simulink model "ModelTest"  (R2018b)
settings: Solver=ode1  StartTime=0.0  StopTime=50.0  FixedStep=0.001  RelTol=1e-3
undefined symbols (not defined in the file): env, sim, steer, vehicle
libraries: simulink x8, dspsrcs4 x1
settings Model: Creator=ogihara  LastModifiedBy=ogihara

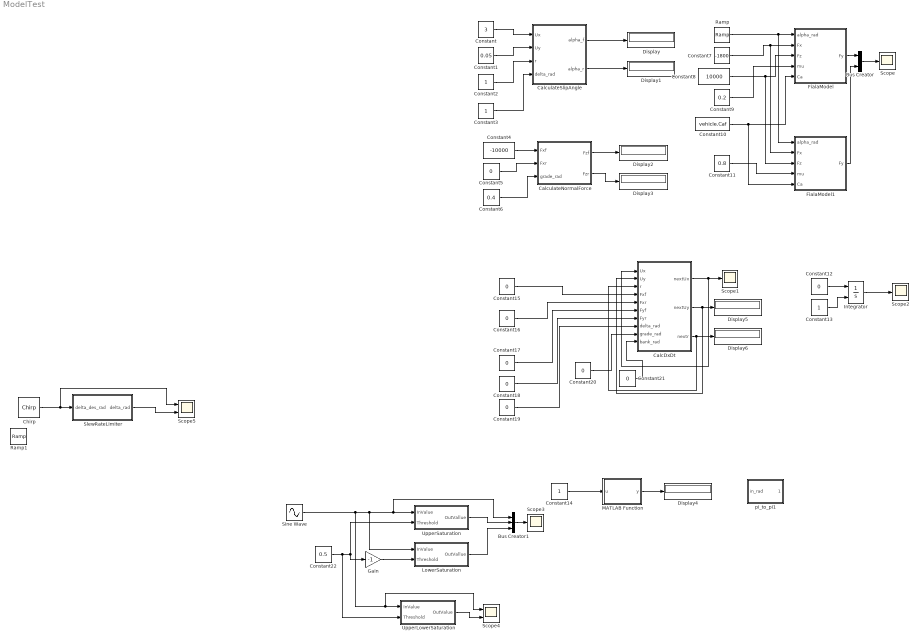
== system ModelTest ==
  Bus Creator : BusCreator  Inputs=2
  Bus Creator1 : BusCreator  Inputs=3
  CalcDxDt : Subsystem
  CalculateNormalForce : Subsystem
  CalculateSlipAngle : Subsystem
  Chirp : dspsrcs4/Chirp  sweep=Linear  mode=Unidirectional  f0=0.1  f1=1  t1=100  Tsweep=100  phase=0  Ts=1/1000  spf=1  datatype=Double  OutputFrames=off
      settings: SourceProductName=DSP System Toolbox
  Constant : Constant  Value=3
  Constant1 : Constant  Value=0.05
  Constant10 : Constant  Value=vehicle.Caf
  Constant11 : Constant  Value=0.8
  Constant{5,12,15..21} (9 alike) : Constant  Value=0
  Constant{2..3,13..14} (4 alike) : Constant
  Constant22 : Constant  Value=0.5
  Constant4 : Constant  Value=-10000
  Constant6 : Constant  Value=0.4
  Constant7 : Constant  Value=-1800
  Constant8 : Constant  Value=10000
  Constant9 : Constant  Value=0.2
  Display{,1..6} (7 alike) : Display
  FialaModel : Subsystem
  FialaModel1 : Subsystem
  Gain : Gain  Gain=-1
  Integrator : Integrator  InitialConditionSource=external
  LowerSaturation : Subsystem
  MATLAB Function : MATLAB Function  TreatAsAtomicUnit=on
  Ramp : simulink/Sources/Ramp  slope=0.1  start=0  InitialOutput=-0.5
  Ramp1 : simulink/Sources/Ramp  slope=1  start=0  InitialOutput=0
  Scope{,1..3} (4 alike) : Scope
  Scope4 : Scope  NumInputPorts=2
  Scope5 : Scope  NumInputPorts=2
  Sine Wave : Sin  SampleTime=0
  SlewRateLimiter : Subsystem
  UpperLowerSaturation : Subsystem
  UpperSaturation : Subsystem
  pi_to_pi1 : Subsystem
  wires:
  CalculateSlipAngle/2(alpha_r) -> Display1/1
  CalculateSlipAngle/1(alpha_f) -> Display/1
  Constant/1 -> CalculateSlipAngle/1(Ux)
  Constant1/1 -> CalculateSlipAngle/2(Uy)
  Constant2/1 -> CalculateSlipAngle/3(r)
  Constant3/1 -> CalculateSlipAngle/4(delta_rad)
  Constant4/1 -> CalculateNormalForce/1(Fxf)
  Constant5/1 -> CalculateNormalForce/2(Fxr)
  Constant6/1 -> CalculateNormalForce/3(grade_rad)
  CalculateNormalForce/1(Fzf) -> Display2/1
  CalculateNormalForce/2(Fzr) -> Display3/1
  Ramp/1 -> FialaModel1/1(alpha_rad), FialaModel/1(alpha_rad)
  Constant7/1 -> FialaModel1/2(Fx), FialaModel/2(Fx)
  Constant8/1 -> FialaModel1/3(Fz), FialaModel/3(Fz)
  Constant9/1 -> FialaModel/4(mu)
  Constant10/1 -> FialaModel1/5(Ca), FialaModel/5(Ca)
  Constant11/1 -> FialaModel1/4(mu)
  FialaModel/1(Fy) -> Bus Creator/1
  FialaModel1/1(Fy) -> Bus Creator/2
  Bus Creator/1 -> Scope/1
  Constant15/1 -> CalcDxDt/4(Fxf)
  Constant16/1 -> CalcDxDt/5(Fxr)
  Constant17/1 -> CalcDxDt/6(Fyf)
  Constant18/1 -> CalcDxDt/7(Fyr)
  Constant19/1 -> CalcDxDt/8(delta_rad)
  Constant21/1 -> CalcDxDt/10(bank_rad)
  Constant20/1 -> CalcDxDt/9(grade_rad)
  CalcDxDt/3(nextr) -> CalcDxDt/3(r), Display6/1
  CalcDxDt/2(nextUy) -> CalcDxDt/2(Uy), Display5/1
  CalcDxDt/1("nextUx ") -> CalcDxDt/1(Ux), Scope1/1
  Integrator/1 -> Scope2/1
  Constant13/1 -> Integrator/2
  Constant12/1 -> Integrator/1
  MATLAB Function/1(y) -> Display4/1
  Constant14/1 -> MATLAB Function/1(u)
  Sine Wave/1 -> Scope4/1, UpperLowerSaturation/1(InValue), LowerSaturation/1(InValue), Bus Creator1/1, UpperSaturation/1(InValue)
  Constant22/1 -> UpperLowerSaturation/2(Threshold), Gain/1, UpperSaturation/2(Threshold)
  Gain/1 -> LowerSaturation/2(Threshold)
  UpperSaturation/1(OutVallue) -> Bus Creator1/2
  LowerSaturation/1(OutVallue) -> Bus Creator1/3
  Bus Creator1/1 -> Scope3/1
  UpperLowerSaturation/1(OutValue) -> Scope4/2
  Chirp/1 -> Scope5/1, SlewRateLimiter/1(delta_des_rad)
  SlewRateLimiter/1(delta_rad) -> Scope5/2

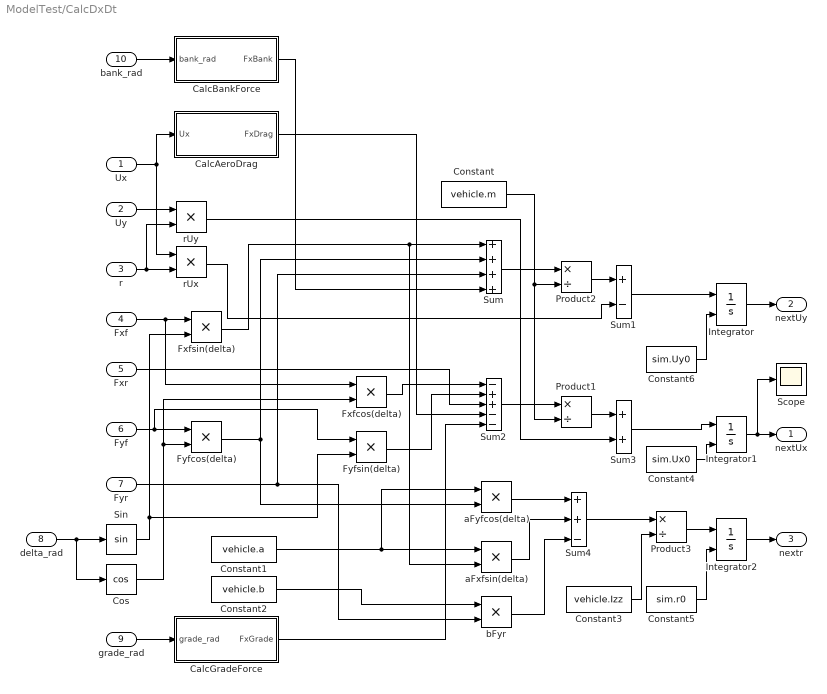
== system ModelTest/CalcDxDt ==
  Ux : Inport
  Uy : Inport  Port=2
  r : Inport  Port=3
  Fxf : Inport  Port=4
  Fxr : Inport  Port=5
  Fyf : Inport  Port=6
  Fyr : Inport  Port=7
  delta_rad : Inport  Port=8
  grade_rad : Inport  Port=9
  bank_rad : Inport  Port=10
  CalcAeroDrag : Subsystem
  CalcBankForce : Subsystem
  CalcGradeForce : Subsystem
  Constant : Constant  Value=vehicle.m
  Constant1 : Constant  Value=vehicle.a
  Constant2 : Constant  Value=vehicle.b
  Constant3 : Constant  Value=vehicle.Izz
  Constant4 : Constant  Value=sim.Ux0
  Constant5 : Constant  Value=sim.r0
  Constant6 : Constant  Value=sim.Uy0
  Cos : Trigonometry  Operator=cos
  Fxfcos(delta) : Product
  Fxfsin(delta) : Product
  Fyfcos(delta) : Product
  Fyfsin(delta) : Product
  Integrator : Integrator  InitialConditionSource=external
  Integrator1 : Integrator  InitialConditionSource=external
  Integrator2 : Integrator  InitialConditionSource=external  InitialCondition=sim.r0
  Product1 : Product  Inputs=*/
  Product2 : Product  Inputs=*/
  Product3 : Product  Inputs=*/
  Scope : Scope
  Sin : Trigonometry
  Sum : Sum  Inputs=++++
  Sum1 : Sum  Inputs=+-
  Sum2 : Sum  Inputs=-++--
  Sum3 : Sum
  Sum4 : Sum  Inputs=++-
  aFxfsin(delta) : Product
  aFyfcos(delta) : Product
  bFyr : Product
  rUx : Product
  rUy : Product
  "nextUx " : Outport
  nextUy : Outport  Port=2
  nextr : Outport  Port=3
  wires:
  delta_rad/1 -> Cos/1, Sin/1
  Fyf/1 -> Fyfsin(delta)/1, Fyfcos(delta)/1
  Cos/1 -> Fxfcos(delta)/2, Fyfcos(delta)/2
  Fxf/1 -> Fxfcos(delta)/1, Fxfsin(delta)/1
  Sin/1 -> Fyfsin(delta)/2, Fxfsin(delta)/2
  Fxfsin(delta)/1 -> Sum/1, aFxfsin(delta)/2
  Fyfcos(delta)/1 -> aFyfcos(delta)/2, Sum/2
  Fyr/1 -> bFyr/2, Sum/3
  grade_rad/1 -> CalcGradeForce/1(grade_rad)
  Constant/1 -> Product1/2, Product2/2
  Sum/1 -> Product2/1
  r/1 -> rUx/2, rUy/2
  Ux/1 -> CalcAeroDrag/1(Ux), rUx/1
  Product2/1 -> Sum1/1
  Sum1/1 -> Integrator/1
  rUx/1 -> Sum1/2
  Uy/1 -> rUy/1
  bank_rad/1 -> CalcBankForce/1(bank_rad)
  CalcBankForce/1(FxBank) -> Sum/4
  Fxfcos(delta)/1 -> Sum2/1
  Fyfsin(delta)/1 -> Sum2/2
  Fxr/1 -> Sum2/3
  CalcAeroDrag/1(FxDrag) -> Sum2/4
  CalcGradeForce/1(FxGrade) -> Sum2/5
  Sum3/1 -> Integrator1/1
  Product1/1 -> Sum3/1
  Sum2/1 -> Product1/1
  rUy/1 -> Sum3/2
  Constant1/1 -> aFxfsin(delta)/1, aFyfcos(delta)/1
  Constant2/1 -> bFyr/1
  aFyfcos(delta)/1 -> Sum4/1
  aFxfsin(delta)/1 -> Sum4/2
  bFyr/1 -> Sum4/3
  Constant3/1 -> Product3/2
  Sum4/1 -> Product3/1
  Product3/1 -> Integrator2/1
  Integrator/1 -> nextUy/1
  Integrator1/1 -> Scope/1, "nextUx "/1
  Integrator2/1 -> nextr/1
  Constant4/1 -> Integrator1/2
  Constant5/1 -> Integrator2/2
  Constant6/1 -> Integrator/2

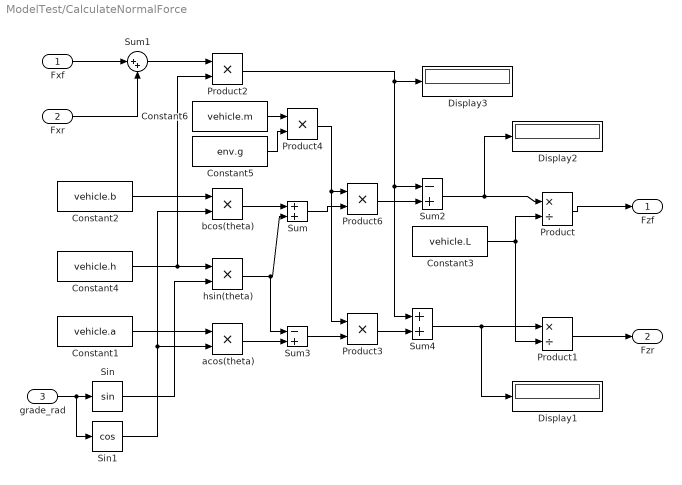
== system ModelTest/CalculateNormalForce ==
  Fxf : Inport
  Fxr : Inport  Port=2
  grade_rad : Inport  Port=3
  Constant1 : Constant  Value=vehicle.a
  Constant2 : Constant  Value=vehicle.b
  Constant3 : Constant  Value=vehicle.L
  Constant4 : Constant  Value=vehicle.h
  Constant5 : Constant  Value=env.g
  Constant6 : Constant  Value=vehicle.m
  Display1 : Display
  Display2 : Display
  Display3 : Display
  Product : Product  Inputs=*/
  Product1 : Product  Inputs=*/
  Product{2..4,6} (4 alike) : Product
  Sin : Trigonometry
  Sin1 : Trigonometry  Operator=cos
  Sum : Sum
  Sum1 : Sum  Inputs=|++
  Sum2 : Sum  Inputs=-+
  Sum3 : Sum  Inputs=-+
  Sum4 : Sum
  acos(theta) : Product
  bcos(theta) : Product
  hsin(theta) : Product
  Fzf : Outport
  Fzr : Outport  Port=2
  wires:
  grade_rad/1 -> Sin1/1, Sin/1
  Constant2/1 -> bcos(theta)/1
  Sin1/1 -> bcos(theta)/2, acos(theta)/2
  Constant1/1 -> acos(theta)/1
  Sin/1 -> hsin(theta)/2
  bcos(theta)/1 -> Sum/1
  hsin(theta)/1 -> Sum3/1, Sum/2
  Sum/1 -> Product6/2
  Fxf/1 -> Sum1/1
  Fxr/1 -> Sum1/2
  Constant4/1 -> Product2/2, hsin(theta)/1
  Sum1/1 -> Product2/1
  Product6/1 -> Sum2/2
  Product2/1 -> Display3/1, Sum4/1, Sum2/1
  Sum2/1 -> Display2/1, Product/1
  Product/1 -> Fzf/1
  acos(theta)/1 -> Sum3/2
  Sum4/1 -> Display1/1, Product1/1
  Product3/1 -> Sum4/2
  Sum3/1 -> Product3/2
  Product1/1 -> Fzr/1
  Constant6/1 -> Product4/1
  Constant5/1 -> Product4/2
  Product4/1 -> Product3/1, Product6/1
  Constant3/1 -> Product1/2, Product/2

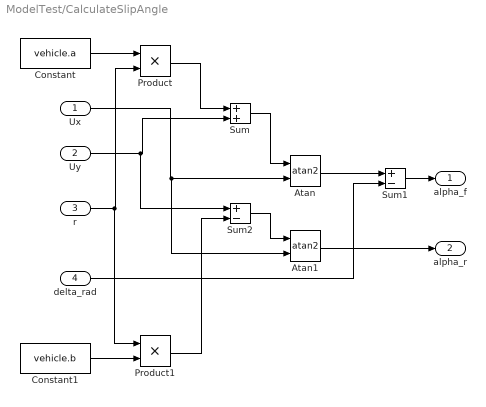
== system ModelTest/CalculateSlipAngle ==
  Ux : Inport
  Uy : Inport  Port=2
  r : Inport  Port=3
  delta_rad : Inport  Port=4
  Atan : Trigonometry  Operator=atan2
  Atan1 : Trigonometry  Operator=atan2
  Constant : Constant  Value=vehicle.a
  Constant1 : Constant  Value=vehicle.b
  Product : Product
  Product1 : Product
  Sum : Sum
  Sum1 : Sum  Inputs=+-
  Sum2 : Sum  Inputs=+-
  alpha_f : Outport
  alpha_r : Outport  Port=2
  wires:
  Constant/1 -> Product/1
  r/1 -> Product1/1, Product/2
  Constant1/1 -> Product1/2
  Ux/1 -> Atan1/2, Atan/2
  Uy/1 -> Sum2/1, Sum/2
  Product/1 -> Sum/1
  Sum/1 -> Atan/1
  delta_rad/1 -> Sum1/2
  Atan/1 -> Sum1/1
  Sum1/1 -> alpha_f/1
  Product1/1 -> Sum2/2
  Sum2/1 -> Atan1/1
  Atan1/1 -> alpha_r/1

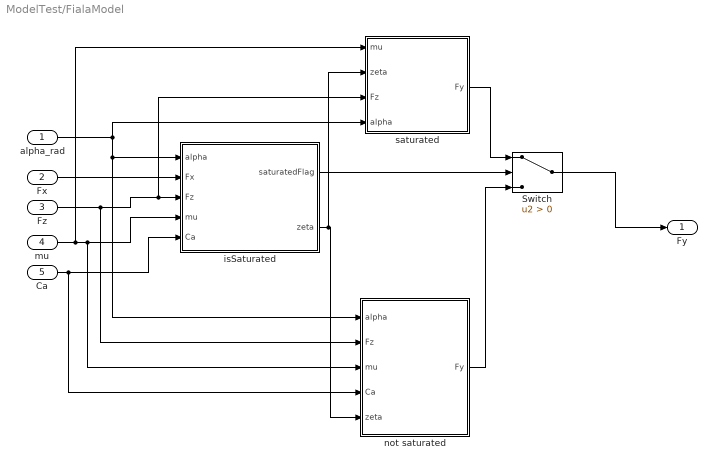
== system ModelTest/FialaModel ==
  alpha_rad : Inport
  Fx : Inport  Port=2
  Fz : Inport  Port=3
  mu : Inport  Port=4
  Ca : Inport  Port=5
  Switch : Switch  Criteria=u2 > Threshold
  isSaturated : Subsystem
  not saturated : Subsystem
  saturated : Subsystem
  Fy : Outport
  wires:
  Switch/1 -> Fy/1
  alpha_rad/1 -> not saturated/1(alpha), isSaturated/1(alpha), saturated/4(alpha)
  Fx/1 -> isSaturated/2(Fx)
  Fz/1 -> not saturated/2(Fz), saturated/3(Fz), isSaturated/3(Fz)
  mu/1 -> saturated/1(mu), not saturated/3(mu), isSaturated/4(mu)
  Ca/1 -> not saturated/4(Ca), isSaturated/5(Ca)
  isSaturated/1(saturatedFlag) -> Switch/2
  saturated/1(Fy) -> Switch/1
  not saturated/1(Fy) -> Switch/3
  isSaturated/2(zeta) -> saturated/2(zeta), not saturated/5(zeta)

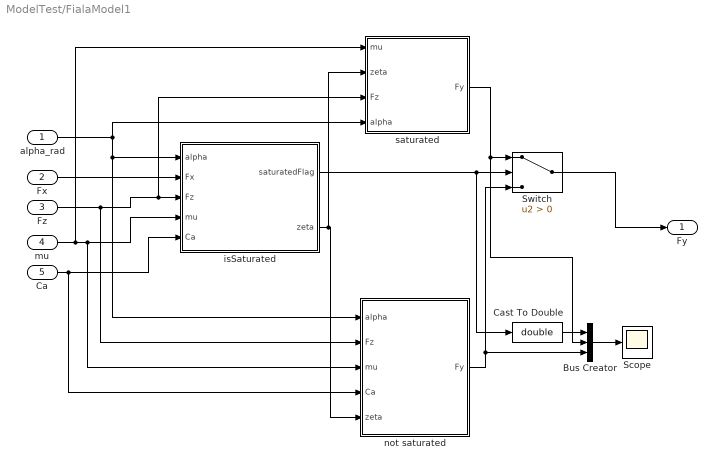
== system ModelTest/FialaModel1 ==
  alpha_rad : Inport
  Fx : Inport  Port=2
  Fz : Inport  Port=3
  mu : Inport  Port=4
  Ca : Inport  Port=5
  Bus Creator : BusCreator  Inputs=3
  Cast To Double : DataTypeConversion  OutDataTypeStr=double
  Scope : Scope
  Switch : Switch  Criteria=u2 > Threshold
  isSaturated : Subsystem
  not saturated : Subsystem
  saturated : Subsystem
  Fy : Outport
  wires:
  Switch/1 -> Fy/1
  alpha_rad/1 -> not saturated/1(alpha), isSaturated/1(alpha), saturated/4(alpha)
  Fx/1 -> isSaturated/2(Fx)
  Fz/1 -> not saturated/2(Fz), saturated/3(Fz), isSaturated/3(Fz)
  mu/1 -> saturated/1(mu), not saturated/3(mu), isSaturated/4(mu)
  Ca/1 -> not saturated/4(Ca), isSaturated/5(Ca)
  isSaturated/1(saturatedFlag) -> Cast To Double/1, Switch/2
  saturated/1(Fy) -> Bus Creator/2, Switch/1
  not saturated/1(Fy) -> Bus Creator/3, Switch/3
  isSaturated/2(zeta) -> saturated/2(zeta), not saturated/5(zeta)
  Bus Creator/1 -> Scope/1
  Cast To Double/1 -> Bus Creator/1

== system ModelTest/LowerSaturation ==
  note: If InValue is smaller than Threshold, Then OutValue is Threshold.
      | Else, OutValue is InValue.
  InValue : Inport
  Threshold : Inport  Port=2
  Compare To Zero : simulink/Logic and Bit Operations/Compare To Zero  relop=>  OutDataTypeStr=boolean
  Minus : Sum  Inputs=-+
  Switch : Switch  Criteria=u2 > Threshold
  OutVallue : Outport
  wires:
  Threshold/1 -> Switch/1, Minus/2
  InValue/1 -> Minus/1, Switch/3
  Minus/1 -> Compare To Zero/1
  Compare To Zero/1 -> Switch/2
  Switch/1 -> OutVallue/1

== system ModelTest/SlewRateLimiter ==
  delta_des_rad : Inport
  Rate Limiter : RateLimiter  RisingSlewLimit=steer.deltaRateMax_radps  FallingSlewLimit=-steer.deltaRateMax_radps  SampleTimeMode=inherited
  delta_rad : Outport
  wires:
  delta_des_rad/1 -> Rate Limiter/1
  Rate Limiter/1 -> delta_rad/1

== system ModelTest/UpperLowerSaturation ==
  note: Output is within [-Threshold, Threshold]
  InValue : Inport
  Threshold : Inport  Port=2
  Abs : Abs
  Gain : Gain  Gain=-1
  LowerSaturation : Subsystem
  UpperSaturation : Subsystem
  OutValue : Outport
  wires:
  LowerSaturation/1(OutVallue) -> OutValue/1
  Threshold/1 -> Abs/1
  InValue/1 -> UpperSaturation/1(InValue)
  Abs/1 -> Gain/1, UpperSaturation/2(Threshold)
  UpperSaturation/1(OutVallue) -> LowerSaturation/1(InValue)
  Gain/1 -> LowerSaturation/2(Threshold)

== system ModelTest/UpperSaturation ==
  note: If InValue is larger than Threshold, Then OutValue is Threshold.
      | Else, OutValue is InValue.
  InValue : Inport
  Threshold : Inport  Port=2
  Compare To Zero : simulink/Logic and Bit Operations/Compare To Zero  relop=>  OutDataTypeStr=boolean
  Minus : Sum  Inputs=+-
  Switch : Switch  Criteria=u2 > Threshold
  OutVallue : Outport
  wires:
  Threshold/1 -> Switch/1, Minus/2
  InValue/1 -> Switch/3, Minus/1
  Minus/1 -> Compare To Zero/1
  Compare To Zero/1 -> Switch/2
  Switch/1 -> OutVallue/1

== system ModelTest/pi_to_pi1 ==
  in_rad : Inport
  Compare To Constant : simulink/Logic and Bit Operations/Compare To Constant  relop=<=  const=-pi  OutDataTypeStr=boolean
  Compare To Constant1 : simulink/Logic and Bit Operations/Compare To Constant  relop=>  const=pi  OutDataTypeStr=boolean
  Constant : Constant  Value=2*pi
  Minus : Sum  Inputs=+-
  Plus : Sum
  Switch : Switch  Criteria=u2 > Threshold
  Switch1 : Switch  Criteria=u2 > Threshold
  out_rad : Outport
  wires:
  Constant/1 -> Minus/2, Plus/2
  in_rad/1 -> Switch/3, Compare To Constant/1, Minus/1, Plus/1
  Compare To Constant1/1 -> Switch1/2
  Compare To Constant/1 -> Switch/2
  Plus/1 -> Switch/1
  Switch/1 -> Switch1/3, Compare To Constant1/1
  Minus/1 -> Switch1/1
  Switch1/1 -> out_rad/1

== system ModelTest/CalcDxDt/CalcAeroDrag ==
  Ux : Inport
  Constant : Constant  Value=vehicle.Cd0
  Gain : Gain  Gain=vehicle.Cd1
  Gain1 : Gain  Gain=vehicle.Cd2
  Product : Product
  Product1 : Product
  Sign : Signum
  Square : Math  Operator=square  SaturateOnIntegerOverflow=on
  Sum : Sum  Inputs=3
  FxDrag : Outport
  wires:
  Sum/1 -> FxDrag/1
  Gain1/1 -> Product1/2
  Gain/1 -> Sum/2
  Square/1 -> Gain1/1
  Ux/1 -> Gain/1, Square/1, Sign/1
  Product/1 -> Sum/1
  Sign/1 -> Product1/1, Product/2
  Constant/1 -> Product/1
  Product1/1 -> Sum/3

== system ModelTest/CalcDxDt/CalcBankForce ==
  bank_rad : Inport
  Constant : Constant  Value=vehicle.m
  Constant1 : Constant  Value=env.g
  Product : Product  Inputs=3
  Sin : Trigonometry
  FxBank : Outport
  wires:
  bank_rad/1 -> Sin/1
  Sin/1 -> Product/1
  Constant/1 -> Product/2
  Constant1/1 -> Product/3
  Product/1 -> FxBank/1

== system ModelTest/CalcDxDt/CalcGradeForce ==
  grade_rad : Inport
  Constant : Constant  Value=vehicle.m
  Constant1 : Constant  Value=env.g
  Product : Product  Inputs=3
  Sin : Trigonometry
  FxGrade : Outport
  wires:
  grade_rad/1 -> Sin/1
  Sin/1 -> Product/1
  Constant/1 -> Product/2
  Constant1/1 -> Product/3
  Product/1 -> FxGrade/1

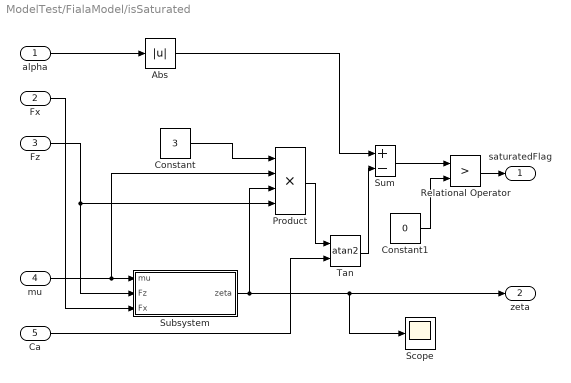
== system ModelTest/FialaModel/isSaturated ==
  alpha : Inport
  Fx : Inport  Port=2
  Fz : Inport  Port=3
  mu : Inport  Port=4
  Ca : Inport  Port=5
  Abs : Abs
  Constant : Constant  Value=3
  Constant1 : Constant  Value=0
  Product : Product  Inputs=4
  Relational Operator : RelationalOperator  Operator=>  OutDataTypeStr=boolean  RndMeth=Simplest
  Scope : Scope
  Subsystem : Subsystem
  Sum : Sum  Inputs=+-
  Tan : Trigonometry  Operator=atan2
  saturatedFlag : Outport
  zeta : Outport  Port=2
  wires:
  Subsystem/1(zeta) -> Scope/1, zeta/1, Product/3
  Product/1 -> Tan/1
  Tan/1 -> Sum/2
  Fx/1 -> Subsystem/3(Fx)
  Fz/1 -> Subsystem/2(Fz), Product/4
  Constant/1 -> Product/1
  mu/1 -> Product/2, Subsystem/1(mu)
  Ca/1 -> Tan/2
  Abs/1 -> Sum/1
  alpha/1 -> Abs/1
  Sum/1 -> Relational Operator/1
  Constant1/1 -> Relational Operator/2
  Relational Operator/1 -> saturatedFlag/1

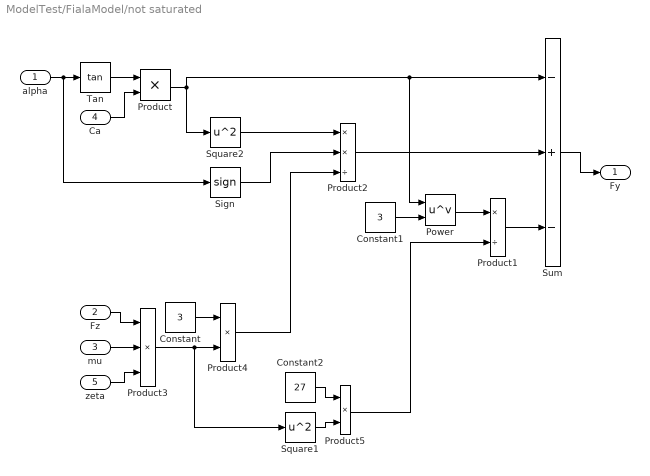
== system ModelTest/FialaModel/not saturated ==
  alpha : Inport
  Fz : Inport  Port=2
  mu : Inport  Port=3
  Ca : Inport  Port=4
  zeta : Inport  Port=5
  Constant : Constant  Value=3
  Constant1 : Constant  Value=3
  Constant2 : Constant  Value=27
  Power : Math  Operator=pow  SaturateOnIntegerOverflow=on
  Product : Product
  Product1 : Product  Inputs=*/
  Product2 : Product  Inputs=**/
  Product3 : Product  Inputs=***
  Product4 : Product
  Product5 : Product
  Sign : Signum
  Square1 : Math  Operator=square  SaturateOnIntegerOverflow=on
  Square2 : Math  Operator=square  SaturateOnIntegerOverflow=on
  Sum : Sum  Inputs=-+-
  Tan : Trigonometry  Operator=tan
  Fy : Outport
  wires:
  Sum/1 -> Fy/1
  alpha/1 -> Sign/1, Tan/1
  Tan/1 -> Product/1
  Ca/1 -> Product/2
  Product/1 -> Square2/1, Power/1, Sum/1
  Square2/1 -> Product2/1
  Product2/1 -> Sum/2
  Fz/1 -> Product3/1
  mu/1 -> Product3/2
  zeta/1 -> Product3/3
  Product3/1 -> Square1/1, Product4/2
  Constant/1 -> Product4/1
  Product4/1 -> Product2/3
  Sign/1 -> Product2/2
  Constant2/1 -> Product5/1
  Square1/1 -> Product5/2
  Constant1/1 -> Power/2
  Power/1 -> Product1/1
  Product5/1 -> Product1/2
  Product1/1 -> Sum/3

== system ModelTest/FialaModel/saturated ==
  mu : Inport
  zeta : Inport  Port=2
  Fz : Inport  Port=3
  alpha : Inport  Port=4
  Gain : Gain  Gain=-1
  Product : Product  Inputs=4
  Sign : Signum
  Fy : Outport
  wires:
  alpha/1 -> Sign/1
  Product/1 -> Gain/1
  Gain/1 -> Fy/1
  mu/1 -> Product/1
  zeta/1 -> Product/2
  Fz/1 -> Product/3
  Sign/1 -> Product/4

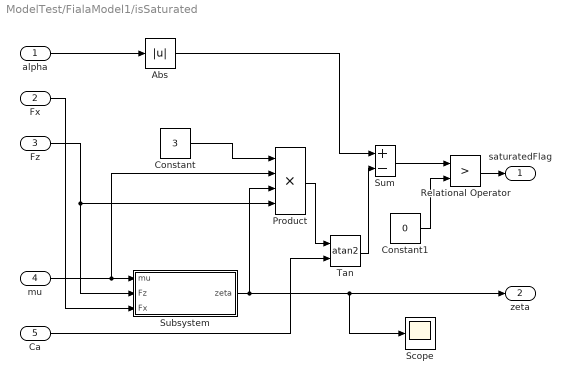
== system ModelTest/FialaModel1/isSaturated ==
  alpha : Inport
  Fx : Inport  Port=2
  Fz : Inport  Port=3
  mu : Inport  Port=4
  Ca : Inport  Port=5
  Abs : Abs
  Constant : Constant  Value=3
  Constant1 : Constant  Value=0
  Product : Product  Inputs=4
  Relational Operator : RelationalOperator  Operator=>  OutDataTypeStr=boolean  RndMeth=Simplest
  Scope : Scope
  Subsystem : Subsystem
  Sum : Sum  Inputs=+-
  Tan : Trigonometry  Operator=atan2
  saturatedFlag : Outport
  zeta : Outport  Port=2
  wires:
  Subsystem/1(zeta) -> Scope/1, zeta/1, Product/3
  Product/1 -> Tan/1
  Tan/1 -> Sum/2
  Fx/1 -> Subsystem/3(Fx)
  Fz/1 -> Subsystem/2(Fz), Product/4
  Constant/1 -> Product/1
  mu/1 -> Product/2, Subsystem/1(mu)
  Ca/1 -> Tan/2
  Abs/1 -> Sum/1
  alpha/1 -> Abs/1
  Sum/1 -> Relational Operator/1
  Constant1/1 -> Relational Operator/2
  Relational Operator/1 -> saturatedFlag/1

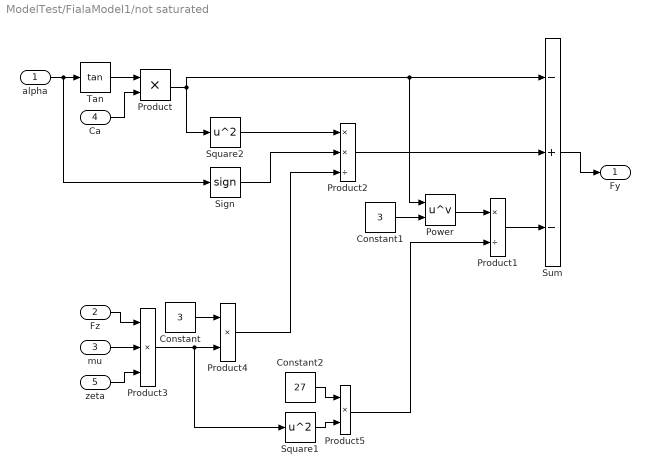
== system ModelTest/FialaModel1/not saturated ==
  alpha : Inport
  Fz : Inport  Port=2
  mu : Inport  Port=3
  Ca : Inport  Port=4
  zeta : Inport  Port=5
  Constant : Constant  Value=3
  Constant1 : Constant  Value=3
  Constant2 : Constant  Value=27
  Power : Math  Operator=pow  SaturateOnIntegerOverflow=on
  Product : Product
  Product1 : Product  Inputs=*/
  Product2 : Product  Inputs=**/
  Product3 : Product  Inputs=***
  Product4 : Product
  Product5 : Product
  Sign : Signum
  Square1 : Math  Operator=square  SaturateOnIntegerOverflow=on
  Square2 : Math  Operator=square  SaturateOnIntegerOverflow=on
  Sum : Sum  Inputs=-+-
  Tan : Trigonometry  Operator=tan
  Fy : Outport
  wires:
  Sum/1 -> Fy/1
  alpha/1 -> Sign/1, Tan/1
  Tan/1 -> Product/1
  Ca/1 -> Product/2
  Product/1 -> Square2/1, Power/1, Sum/1
  Square2/1 -> Product2/1
  Product2/1 -> Sum/2
  Fz/1 -> Product3/1
  mu/1 -> Product3/2
  zeta/1 -> Product3/3
  Product3/1 -> Square1/1, Product4/2
  Constant/1 -> Product4/1
  Product4/1 -> Product2/3
  Sign/1 -> Product2/2
  Constant2/1 -> Product5/1
  Square1/1 -> Product5/2
  Constant1/1 -> Power/2
  Power/1 -> Product1/1
  Product5/1 -> Product1/2
  Product1/1 -> Sum/3

== system ModelTest/FialaModel1/saturated ==
  mu : Inport
  zeta : Inport  Port=2
  Fz : Inport  Port=3
  alpha : Inport  Port=4
  Gain : Gain  Gain=-1
  Product : Product  Inputs=4
  Sign : Signum
  Fy : Outport
  wires:
  alpha/1 -> Sign/1
  Product/1 -> Gain/1
  Gain/1 -> Fy/1
  mu/1 -> Product/1
  zeta/1 -> Product/2
  Fz/1 -> Product/3
  Sign/1 -> Product/4

== system ModelTest/UpperLowerSaturation/LowerSaturation ==
  note: If InValue is smaller than Threshold, Then OutValue is Threshold.
      | Else, OutValue is InValue.
  InValue : Inport
  Threshold : Inport  Port=2
  Compare To Zero : simulink/Logic and Bit Operations/Compare To Zero  relop=>  OutDataTypeStr=boolean
  Minus : Sum  Inputs=-+
  Switch : Switch  Criteria=u2 > Threshold
  OutVallue : Outport
  wires:
  Threshold/1 -> Switch/1, Minus/2
  InValue/1 -> Minus/1, Switch/3
  Minus/1 -> Compare To Zero/1
  Compare To Zero/1 -> Switch/2
  Switch/1 -> OutVallue/1

== system ModelTest/UpperLowerSaturation/UpperSaturation ==
  note: If InValue is larger than Threshold, Then OutValue is Threshold.
      | Else, OutValue is InValue.
  InValue : Inport
  Threshold : Inport  Port=2
  Compare To Zero : simulink/Logic and Bit Operations/Compare To Zero  relop=>  OutDataTypeStr=boolean
  Minus : Sum  Inputs=+-
  Switch : Switch  Criteria=u2 > Threshold
  OutVallue : Outport
  wires:
  Threshold/1 -> Switch/1, Minus/2
  InValue/1 -> Switch/3, Minus/1
  Minus/1 -> Compare To Zero/1
  Compare To Zero/1 -> Switch/2
  Switch/1 -> OutVallue/1

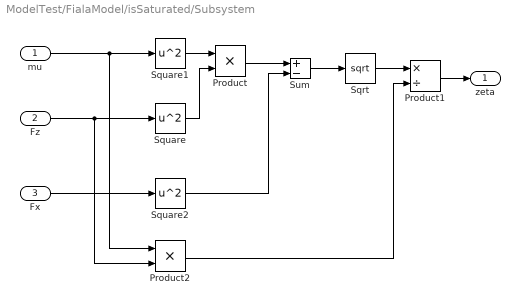
== system ModelTest/FialaModel/isSaturated/Subsystem ==
  mu : Inport
  Fz : Inport  Port=2
  Fx : Inport  Port=3
  Product : Product
  Product1 : Product  Inputs=*/
  Product2 : Product
  Sqrt : Sqrt  SaturateOnIntegerOverflow=on
  Square : Math  Operator=square  SaturateOnIntegerOverflow=on
  Square1 : Math  Operator=square  SaturateOnIntegerOverflow=on
  Square2 : Math  Operator=square  SaturateOnIntegerOverflow=on
  Sum : Sum  Inputs=+-
  zeta : Outport
  wires:
  mu/1 -> Product2/1, Square1/1
  Fz/1 -> Product2/2, Square/1
  Fx/1 -> Square2/1
  Square1/1 -> Product/1
  Square/1 -> Product/2
  Product/1 -> Sum/1
  Square2/1 -> Sum/2
  Sum/1 -> Sqrt/1
  Sqrt/1 -> Product1/1
  Product2/1 -> Product1/2
  Product1/1 -> zeta/1

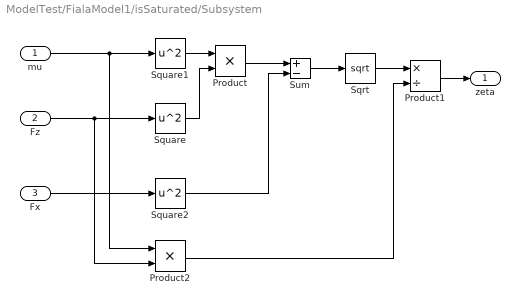
== system ModelTest/FialaModel1/isSaturated/Subsystem ==
  mu : Inport
  Fz : Inport  Port=2
  Fx : Inport  Port=3
  Product : Product
  Product1 : Product  Inputs=*/
  Product2 : Product
  Sqrt : Sqrt  SaturateOnIntegerOverflow=on
  Square : Math  Operator=square  SaturateOnIntegerOverflow=on
  Square1 : Math  Operator=square  SaturateOnIntegerOverflow=on
  Square2 : Math  Operator=square  SaturateOnIntegerOverflow=on
  Sum : Sum  Inputs=+-
  zeta : Outport
  wires:
  mu/1 -> Product2/1, Square1/1
  Fz/1 -> Product2/2, Square/1
  Fx/1 -> Square2/1
  Square1/1 -> Product/1
  Square/1 -> Product/2
  Product/1 -> Sum/1
  Square2/1 -> Sum/2
  Sum/1 -> Sqrt/1
  Sqrt/1 -> Product1/1
  Product2/1 -> Product1/2
  Product1/1 -> zeta/1

== matlab function ModelTest/MATLAB Function ==
  data: u input; y output
function y = fcn(u)

y = 2*u;
